simulink model "SS_elasticoPD_q"  (R2024b)
settings: Solver=ode3  StartTime=0.0  StopTime=tsamplesimulink  FixedStep=0.00001  MaxStep=0.001  RelTol=1e-3  AbsTol=1e-3  EnableMultiTasking=on
undefined symbols (not defined in the file): Ac, Bc, Cc, Dc, Kp, Kv, N
settings Model: Creator=rzotovic  LastModifiedBy=ruizh
settings SolverCC: AutoScaleAbsTol=off  AlgebraicLoopSolver=TrustRegion
settings DataIOCC: SaveFormat=Array  SignalLoggingSaveFormat=ModelDataLogs  SaveOutput=off  SaveTime=off  ReturnWorkspaceOutputs=off
settings OptimizationCC: BlockReduction=off  BooleanDataType=off  ExpressionDepthLimit=2147483647  LifeSpan=inf
settings DebuggingCC: SaveWithParameterizedLinksMsg=none  UnderspecifiedInitializationDetection=Classic  MergeDetectMultiDrivingBlocksExec=none  SignalResolutionControl=TryResolveAllWithWarning  MultiTaskDSMMsg=warning  MultiTaskCondExecSysMsg=none  FcnCallInpInsideContextMsg=warning  UnconnectedInputMsg=warning  UnconnectedOutputMsg=warning  UnconnectedLineMsg=warning  StateNameClashWarn=warning  SFUnexpectedBacktrackingDiag=warning  SFNoUnconditionalDefaultTransitionDiag=warning  SFExecutionAtInitializationDiag=none  ArithmeticOperatorsInVariantConditions=warning
settings HardwareCC: ProdBitPerPointer=32  ProdBitPerSizeT=32  ProdBitPerPtrDiffT=32  ProdLargestAtomicFloat=None  ProdIntDivRoundTo=Undefined  ProdEndianess=Unspecified  ProdWordSize=32  ProdHWDeviceType=32-bit Generic  TargetUnknown=on
settings ModelReferenceCC: EnableRefExpFcnMdlSchedulingChecks=on  PropagateSignalLabelsOutOfModel=off
settings SFSimCC: SimUseLocalCustomCode=off  CustomCodeUndefinedFunction=UseInterfaceOnly
settings RTWCC: RTWUseLocalCustomCode=off  GPUComputeCapability=3.5
settings CodeAppCC: StateflowObjectComments=on
settings GRTTargetCC: TargetLangStandard=C89/C90 (ANSI)  CombineOutputUpdateFcns=off  GRTInterface=on
settings ConfigComp: CovMetricSettings=dw  CovSaveCumulativeToWorkspaceVar=on  CovSaveSingleToWorkspaceVar=on  CovExternalEMLEnable=off  CovSFcnEnable=off

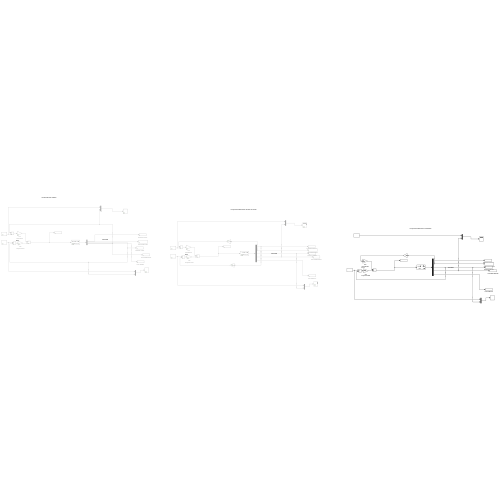
[thumbnail: Simulink's stored preview of the top-level diagram]
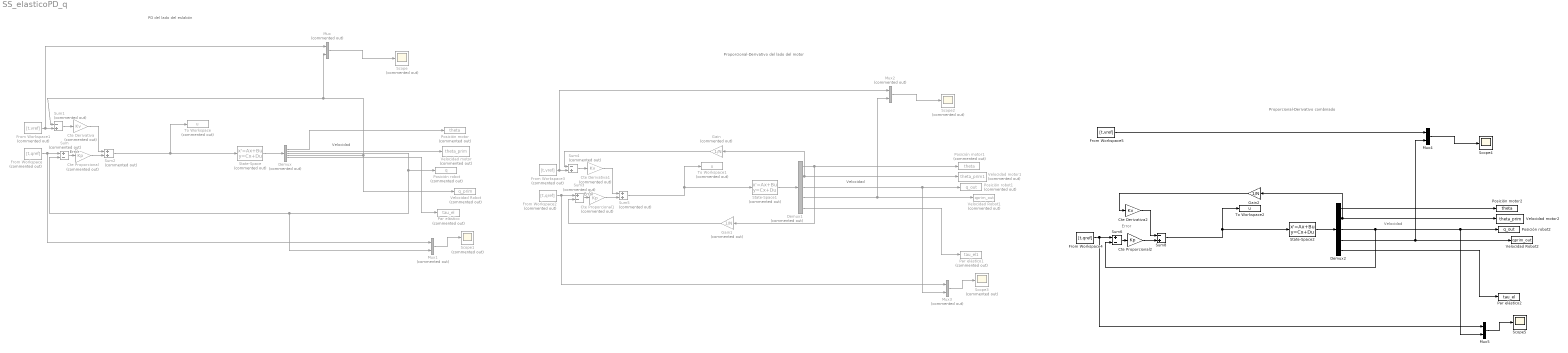
== system SS_elasticoPD_q ==
  note: PD del lado del eslabón
  note: Proporcional-Derivativo del lado del motor
  note: Velocidad
  note: Error
  note: Velocidad
  note: Error
  note: Proporcional-Derivativo combinado
  note: Error
  note: Velocidad
  Cte Derivativa : Gain  Commented=on  Gain=Kv  SaturateOnIntegerOverflow=on  OutDataTypeStr=Inherit: Same as input  ParamDataTypeStr=Inherit: Same as input
  Cte Derivativa1 : Gain  Commented=on  Gain=Kv  SaturateOnIntegerOverflow=on  OutDataTypeStr=Inherit: Same as input  ParamDataTypeStr=Inherit: Same as input
  Cte Derivativa2 : Gain  Gain=Kv  SaturateOnIntegerOverflow=on  OutDataTypeStr=Inherit: Same as input  ParamDataTypeStr=Inherit: Same as input
  Cte Proporcional : Gain  Commented=on  Gain=Kp  SaturateOnIntegerOverflow=on  OutDataTypeStr=Inherit: Same as input  ParamDataTypeStr=Inherit: Same as input
  Cte Proporcional1 : Gain  Commented=on  Gain=Kp  SaturateOnIntegerOverflow=on  OutDataTypeStr=Inherit: Same as input  ParamDataTypeStr=Inherit: Same as input
  Cte Proporcional2 : Gain  Gain=Kp  SaturateOnIntegerOverflow=on  OutDataTypeStr=Inherit: Same as input  ParamDataTypeStr=Inherit: Same as input
  Demux : Demux  Commented=on  Outputs=5
  Demux1 : Demux  Commented=on  Outputs=5
  Demux2 : Demux  Outputs=5
  From Workspace : FromWorkspace  Commented=on  VariableName=[t,qref]  SampleTime=0.00001  ZeroCross=off
  From Workspace1 : FromWorkspace  Commented=on  VariableName=[t,vref]  SampleTime=0.00001  ZeroCross=off
  From Workspace2 : FromWorkspace  Commented=on  VariableName=[t,qref]  SampleTime=0.00001  ZeroCross=off
  From Workspace3 : FromWorkspace  Commented=on  VariableName=[t,vref]  SampleTime=0.00001  ZeroCross=off
  From Workspace4 : FromWorkspace  VariableName=[t,qref]  SampleTime=0.00001  ZeroCross=off
  From Workspace5 : FromWorkspace  VariableName=[t,vref]  SampleTime=0.00001  ZeroCross=off
  Gain : Gain  Commented=on  Gain=1/N
  Gain1 : Gain  Commented=on  Gain=1/N
  Gain2 : Gain  Gain=1/N
  Mux{,1..3} (4 alike) : Mux  Commented=on  Inputs=2
  Mux4 : Mux  Inputs=2
  Mux5 : Mux  Inputs=2
  Par elástico : ToWorkspace  Commented=on  VariableName=tau_el
      settings: MaxDataPoints=samplesimulink
  Par elástico1 : ToWorkspace  Commented=on  VariableName=tau_el1
      settings: MaxDataPoints=samplesimulink
  Par elástico2 : ToWorkspace  VariableName=tau_el
      settings: MaxDataPoints=samplesimulink
  Posición motor : ToWorkspace  Commented=on  VariableName=theta
      settings: MaxDataPoints=samplesimulink
  Posición motor1 : ToWorkspace  Commented=on  VariableName=theta
      settings: MaxDataPoints=samplesimulink
  Posición motor2 : ToWorkspace  VariableName=theta
      settings: MaxDataPoints=samplesimulink
  Posición robot : ToWorkspace  Commented=on  VariableName=q
      settings: MaxDataPoints=samplesimulink
  Posición robot1 : ToWorkspace  Commented=on  VariableName=q_out
      settings: MaxDataPoints=samplesimulink
  Posición robot2 : ToWorkspace  VariableName=q_out
      settings: MaxDataPoints=samplesimulink
  Scope{,1..3} (4 alike) : Scope  Commented=on
  Scope4 : Scope
  Scope5 : Scope
  State-Space : StateSpace  Commented=on  A=Ac  B=Bc  C=Cc  D=Dc  InitialCondition=0
  State-Space1 : StateSpace  Commented=on  A=Ac  B=Bc  C=Cc  D=Dc  InitialCondition=0
  State-Space2 : StateSpace  A=Ac  B=Bc  C=Cc  D=Dc  InitialCondition=0
  Sum : Sum  Commented=on  Inputs=+-  InputSameDT=on  SaturateOnIntegerOverflow=on  OutDataTypeStr=Inherit: Same as first input
  Sum1 : Sum  Commented=on  Inputs=-+  InputSameDT=on  SaturateOnIntegerOverflow=on  OutDataTypeStr=Inherit: Same as first input
  Sum2 : Sum  Commented=on  InputSameDT=on  SaturateOnIntegerOverflow=on  OutDataTypeStr=Inherit: Same as first input
  Sum3 : Sum  Commented=on  Inputs=+-  InputSameDT=on  SaturateOnIntegerOverflow=on  OutDataTypeStr=Inherit: Same as first input
  Sum4 : Sum  Commented=on  Inputs=-+  InputSameDT=on  SaturateOnIntegerOverflow=on  OutDataTypeStr=Inherit: Same as first input
  Sum5 : Sum  Commented=on  InputSameDT=on  SaturateOnIntegerOverflow=on  OutDataTypeStr=Inherit: Same as first input
  Sum6 : Sum  Inputs=+-  InputSameDT=on  SaturateOnIntegerOverflow=on  OutDataTypeStr=Inherit: Same as first input
  Sum8 : Sum  Inputs=-+  InputSameDT=on  SaturateOnIntegerOverflow=on  OutDataTypeStr=Inherit: Same as first input
  To Workspace : ToWorkspace  Commented=on  VariableName=u
      settings: MaxDataPoints=11333
  To Workspace1 : ToWorkspace  Commented=on  VariableName=u
      settings: MaxDataPoints=11333
  To Workspace2 : ToWorkspace  VariableName=u
      settings: MaxDataPoints=11333
  Velocidad Robot : ToWorkspace  Commented=on  VariableName=q_prim
      settings: MaxDataPoints=samplesimulink
  Velocidad Robot1 : ToWorkspace  Commented=on  VariableName=qprim_out
      settings: MaxDataPoints=samplesimulink
  Velocidad Robot2 : ToWorkspace  VariableName=qprim_out
      settings: MaxDataPoints=samplesimulink
  Velocidad motor : ToWorkspace  Commented=on  VariableName=theta_prim
      settings: MaxDataPoints=samplesimulink
  Velocidad motor1 : ToWorkspace  Commented=on  VariableName=theta_prim1
      settings: MaxDataPoints=samplesimulink
  Velocidad motor2 : ToWorkspace  VariableName=theta_prim
      settings: MaxDataPoints=samplesimulink
  wires:
  Sum2/1 -> To Workspace/1, State-Space/1
  Sum/1 -> Cte Proporcional/1
  Sum1/1 -> Cte Derivativa/1
  From Workspace1/1 -> Mux/1, Sum1/2
  Cte Proporcional/1 -> Sum2/2
  Cte Derivativa/1 -> Sum2/1
  State-Space/1 -> Demux/1
  Demux/1 -> Posición motor/1
  Demux/2 -> Velocidad motor/1
  Demux/4 -> Velocidad Robot/1, Mux/2, Sum1/1
  Mux/1 -> Scope/1
  Mux1/1 -> Scope1/1
  Demux/3 -> Mux1/2, Sum/2, Posición robot/1
  From Workspace/1 -> Mux1/1, Sum/1
  Demux/5 -> Par elástico/1
  Sum5/1 -> To Workspace1/1, State-Space1/1
  Sum3/1 -> Cte Proporcional1/1
  State-Space1/1 -> Demux1/1
  Cte Proporcional1/1 -> Sum5/2
  Mux2/1 -> Scope2/1
  Demux1/4 -> Velocidad Robot1/1, Mux2/2
  From Workspace2/1 -> Mux3/1, Sum3/1
  Demux1/3 -> Mux3/2, Posición robot1/1
  Sum4/1 -> Cte Derivativa1/1
  Mux3/1 -> Scope3/1
  Demux1/1 -> Gain1/1, Posición motor1/1
  From Workspace3/1 -> Mux2/1, Sum4/2
  Cte Derivativa1/1 -> Sum5/1
  Demux1/2 -> Gain/1, Velocidad motor1/1
  Demux1/5 -> Par elástico1/1
  Gain/1 -> Sum4/1
  Gain1/1 -> Sum3/2
  Mux5/1 -> Scope5/1
  Demux2/2 -> Gain2/1, Velocidad motor2/1
  Cte Derivativa2/1 -> Sum8/1
  Demux2/3 -> Sum6/2, Mux5/2, Posición robot2/1
  Gain2/1 -> Cte Derivativa2/1
  Demux2/5 -> Par elástico2/1
  From Workspace4/1 -> Mux5/1, Sum6/1
  Cte Proporcional2/1 -> Sum8/2
  Sum6/1 -> Cte Proporcional2/1
  State-Space2/1 -> Demux2/1
  Sum8/1 -> To Workspace2/1, State-Space2/1
  Mux4/1 -> Scope4/1
  Demux2/1 -> Posición motor2/1
  Demux2/4 -> Velocidad Robot2/1, Mux4/2
  From Workspace5/1 -> Mux4/1
